simulink model "time_opt_control_of_harmonic_oscillator"  (R2023b)
settings: Solver=VariableStepAuto  StartTime=0.0  StopTime=230  MaxStep=1e-4  MinStep=1e-5  RelTol=1e-3
settings Model: SimulationMode=rapid-accelerator  Creator=91798  LastModifiedBy=91798

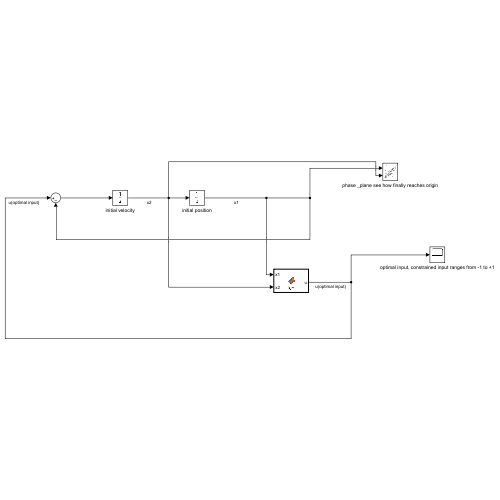
[thumbnail: Simulink's stored preview of the top-level diagram]
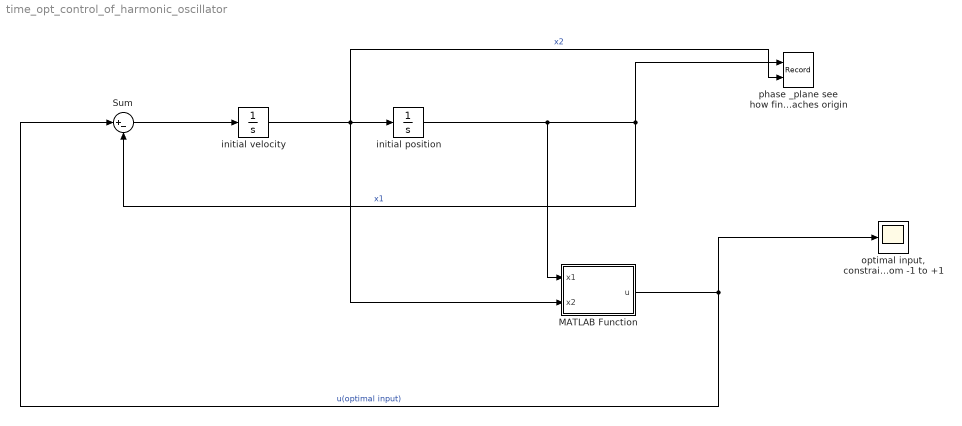
== system time_opt_control_of_harmonic_oscillator ==
  MATLAB Function : MATLAB Function  TreatAsAtomicUnit=on
  Sum : Sum  Inputs=|+-
  initial position : Integrator  InitialCondition=99
  initial velocity : Integrator  InitialCondition=80
  "optimal input, constrained input ranges from -1 to +1" : Scope
  phase _plane see how finally reaches origin : Record  FileSettingsInternal="{\"entries\":[{\"content\":{\"excelSettings\":{\"content\":{},\"type\":\"Streamout.ExcelSettings\"}},\"type\":\"Streamout.FileSettingStorage\",\"uuid\":\"\"}],\"packageUris\":[\"http:\\/\\/schema.mathworks.com\\/mf0\\/streamout_blocks\\/R2020a\"],\"version\":\"1.0\"}"  Layout=[1 1]  SignalsInternal="{\"entries\":[{\"content\":{\"signals\":[{\"content\":{\"blockPath\":[],\"dimensions\":[1],\"domain\":\"\",\"lineColor\":\"#64d413\",\"plots\":[1],\"port\":1,\"signalID\":8,\"signalName\":\"x1\"},\"type\":\"RecordBlkView.Signal\",\"uuid\":\"\"},{\"content\":{\"blockPath\":[],\"dimensions\":[1],\"domain\":\"\",\"lineColor\":\"#ff13a6\",\"plots\":[1],\"port\":2,\"signalID\":11,\"signalName\":\"x2\"},\"type\":\"RecordBlkView.Signal\",\"uuid\":\"\"}]},\"type\":\"RecordBlkView.InputSignals\",\"uuid\":\"\"}],\"packageUris\":[\"http:\\/\\/schema.mathworks.com\\/mf0\\/streamout_blocks\\/R2020a\"],\"version\":\"1.0\"}"  VisualizationBindings="{\"xyplotplugin\":{\"info\":[{\"series\":[{\"bindingParametersList\":[{\"parameter\":\"Y-Axis\",\"signalID\":11,\"signalName\":\"x2\"},{\"parameter\":\"X-Axis\",\"signalID\":8,\"signalName\":\"x1\"}],\"seriesID\":55547}],\"subplotID\":1}]}}"  CompatibilityTag=XY  st=-1
  wires:
  initial velocity/1 -> MATLAB Function/2(x2), phase _plane see how finally reaches origin/2, initial position/1  "x2"
  initial position/1 -> MATLAB Function/1(x1), Sum/2, phase _plane see how finally reaches origin/1  "x1"
  Sum/1 -> initial velocity/1
  MATLAB Function/1(u) -> Sum/1, "optimal input, constrained input ranges from -1 to +1"/1  "u(optimal input)"

== matlab function time_opt_control_of_harmonic_oscillator/MATLAB Function ==
  data: x1 input; u output; x2 input
function u = fcn(x1,x2)

% switching logic 

if ( x2>1 || (x1>0 && x2>0))
    u=-1;

  elseif (x2<-1 || (x1<0 && x2<0))
    u=1;

else n=floor(abs(x1));
   if mod(n,2)==0
    n=n+1;
  end

if (x1<0 && x2>0 && ((x1+n)^2+(x2)^2-1)>0)
   u=-1; 

  elseif (x1>0 && x2<0 && ((x1-n)^2+(x2)^2-1)<0) 
    u=-1;

else u=1;

    end
  end
end
